simulink model "QuadcopterModel"  (R2023b)
settings: Solver=VariableStepAuto  StartTime=0.0  StopTime=200  RelTol=1e-3
values from neighbouring files (symbols this model uses):
  g = 9.81    [QuadcopterParameters.m]
  Ixx = 7.5e-3    (= 0.0075)    [QuadcopterParameters.m]
  Iyy = 7.5e-3    (= 0.0075)    [QuadcopterParameters.m]
  Izz = 1.3e-2    (= 0.013)    [QuadcopterParameters.m]
  Kf = 3.13e-5    (= 3.13e-05)    [QuadcopterParameters.m]
  Km = 7.5e-7    (= 7.5e-07)    [QuadcopterParameters.m]
  l = 0.23    [QuadcopterParameters.m]
  m = 0.65    [QuadcopterParameters.m]
  w1 = 200    [QuadcopterParameters.m]
  w2 = 200    [QuadcopterParameters.m]
  w3 = 10    [QuadcopterParameters.m]
  w4 = 10    [QuadcopterParameters.m]
undefined symbols (not defined in the file or in its folder): magnitude
settings Model: LastModifiedBy=DELL

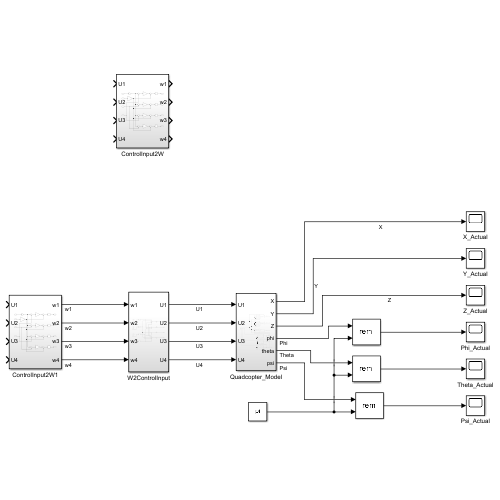
[thumbnail: Simulink's stored preview of the top-level diagram]
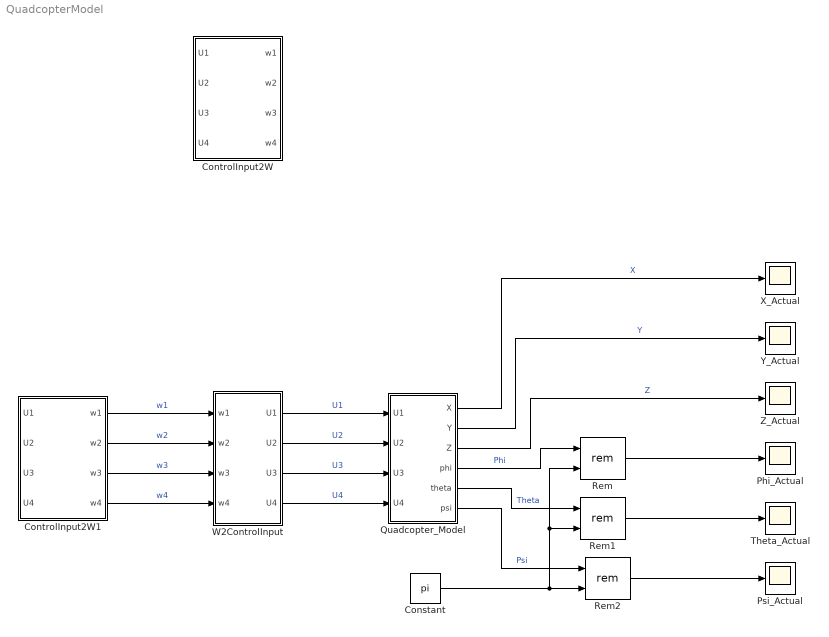
== system QuadcopterModel ==
  Constant : Constant  Value=pi
  ControlInput2W : Subsystem
  ControlInput2W1 : Subsystem
  Phi_Actual : Scope
  Psi_Actual : Scope
  Quadcopter_Model : Subsystem
  Rem : Math  Operator=rem
  Rem1 : Math  Operator=rem
  Rem2 : Math  Operator=rem
  Theta_Actual : Scope
  W2ControlInput : Subsystem
  X_Actual : Scope
  Y_Actual : Scope
  Z_Actual : Scope
  wires:
  W2ControlInput/1(U1) -> Quadcopter_Model/1(U1)  "U1"
  W2ControlInput/4(U4) -> Quadcopter_Model/4(U4)  "U4"
  Quadcopter_Model/3(Z) -> Z_Actual/1  "Z"
  Quadcopter_Model/2(Y) -> Y_Actual/1  "Y"
  Quadcopter_Model/1(X) -> X_Actual/1  "X"
  Constant/1 -> Rem2/2, Rem1/2, Rem/2
  Rem/1 -> Phi_Actual/1
  Rem1/1 -> Theta_Actual/1
  Rem2/1 -> Psi_Actual/1
  Quadcopter_Model/4(phi) -> Rem/1  "Phi"
  Quadcopter_Model/5(theta) -> Rem1/1  "Theta"
  Quadcopter_Model/6(psi) -> Rem2/1  "Psi"
  W2ControlInput/2(U2) -> Quadcopter_Model/2(U2)  "U2"
  W2ControlInput/3(U3) -> Quadcopter_Model/3(U3)  "U3"
  ControlInput2W1/1(w1) -> W2ControlInput/1(w1)  "w1"
  ControlInput2W1/2(w2) -> W2ControlInput/2(w2)  "w2"
  ControlInput2W1/3(w3) -> W2ControlInput/3(w3)  "w3"
  ControlInput2W1/4(w4) -> W2ControlInput/4(w4)  "w4"

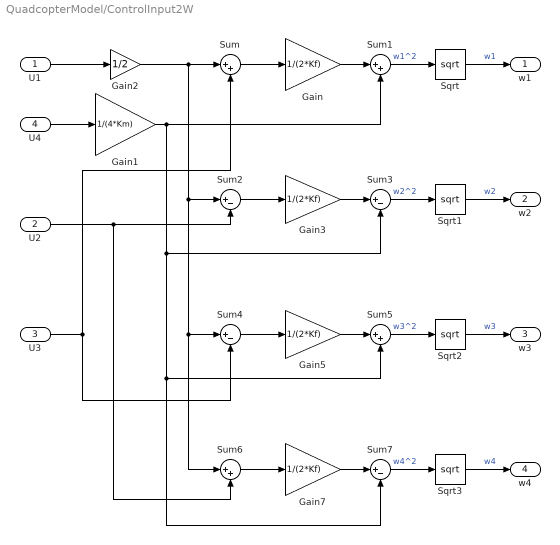
== system QuadcopterModel/ControlInput2W ==
  U1 : Inport
  U2 : Inport  Port=2
  U3 : Inport  Port=3
  U4 : Inport  Port=4
  Gain{,3,5,7} (4 alike) : Gain  Gain=1/(2*Kf)
  Gain1 : Gain  Gain=1/(4*Km)
  Gain2 : Gain  Gain=1/2
  Sqrt{,1..3} (4 alike) : Sqrt
  Sum{,1,5..6} (4 alike) : Sum  Inputs=|++
  Sum{2..4,7} (4 alike) : Sum  Inputs=|+-
  w1 : Outport
  w2 : Outport  Port=2
  w3 : Outport  Port=3
  w4 : Outport  Port=4
  wires:
  Sum7/1 -> Sqrt3/1  "w4^2"
  Gain5/1 -> Sum5/1
  Sum2/1 -> Gain3/1
  Gain/1 -> Sum1/1
  Gain3/1 -> Sum3/1
  Sqrt/1 -> w1/1  "w1"
  Gain7/1 -> Sum7/1
  Sum4/1 -> Gain5/1
  Sqrt1/1 -> w2/1  "w2"
  U2/1 -> Sum2/2, Sum6/2
  Sqrt2/1 -> w3/1  "w3"
  U1/1 -> Gain2/1
  Sqrt3/1 -> w4/1  "w4"
  Sum/1 -> Gain/1
  Gain2/1 -> Sum6/1, Sum4/1, Sum2/1, Sum/1
  Sum3/1 -> Sqrt1/1  "w2^2"
  U3/1 -> Sum/2, Sum4/2
  Sum6/1 -> Gain7/1
  Gain1/1 -> Sum3/2, Sum5/2, Sum7/2, Sum1/2
  Sum1/1 -> Sqrt/1  "w1^2"
  U4/1 -> Gain1/1
  Sum5/1 -> Sqrt2/1  "w3^2"

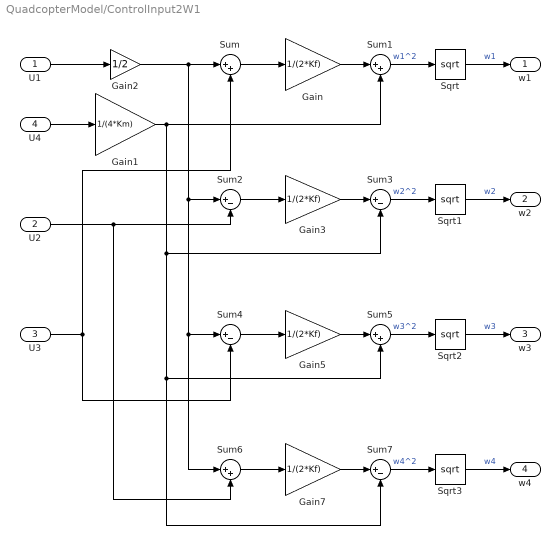
== system QuadcopterModel/ControlInput2W1 ==
  U1 : Inport
  U2 : Inport  Port=2
  U3 : Inport  Port=3
  U4 : Inport  Port=4
  Gain{,3,5,7} (4 alike) : Gain  Gain=1/(2*Kf)
  Gain1 : Gain  Gain=1/(4*Km)
  Gain2 : Gain  Gain=1/2
  Sqrt{,1..3} (4 alike) : Sqrt
  Sum{,1,5..6} (4 alike) : Sum  Inputs=|++
  Sum{2..4,7} (4 alike) : Sum  Inputs=|+-
  w1 : Outport
  w2 : Outport  Port=2
  w3 : Outport  Port=3
  w4 : Outport  Port=4
  wires:
  Sum7/1 -> Sqrt3/1  "w4^2"
  Gain5/1 -> Sum5/1
  Sum2/1 -> Gain3/1
  Gain/1 -> Sum1/1
  Gain3/1 -> Sum3/1
  Sqrt/1 -> w1/1  "w1"
  Gain7/1 -> Sum7/1
  Sum4/1 -> Gain5/1
  Sqrt1/1 -> w2/1  "w2"
  U2/1 -> Sum2/2, Sum6/2
  Sqrt2/1 -> w3/1  "w3"
  U1/1 -> Gain2/1
  Sqrt3/1 -> w4/1  "w4"
  Sum/1 -> Gain/1
  Gain2/1 -> Sum6/1, Sum4/1, Sum2/1, Sum/1
  Sum3/1 -> Sqrt1/1  "w2^2"
  U3/1 -> Sum/2, Sum4/2
  Sum6/1 -> Gain7/1
  Gain1/1 -> Sum3/2, Sum5/2, Sum7/2, Sum1/2
  Sum1/1 -> Sqrt/1  "w1^2"
  U4/1 -> Gain1/1
  Sum5/1 -> Sqrt2/1  "w3^2"

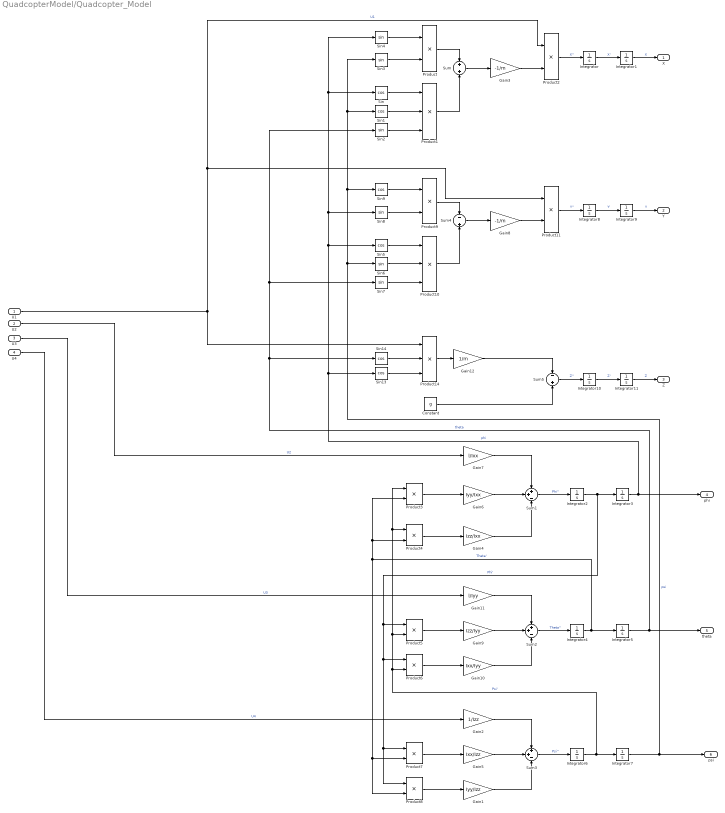
== system QuadcopterModel/Quadcopter_Model ==
  U1 : Inport
  U2 : Inport  Port=2
  U3 : Inport  Port=3
  U4 : Inport  Port=4
  Constant : Constant  Value=g
  Gain1 : Gain  Gain=Iyy/Izz
  Gain10 : Gain  Gain=Ixx/Iyy
  Gain11 : Gain  Gain=l/Iyy
  Gain12 : Gain  Gain=1/m
  Gain2 : Gain  Gain=1/Izz
  Gain3 : Gain  Gain=-1/m
  Gain4 : Gain  Gain=Izz/Ixx
  Gain5 : Gain  Gain=Ixx/Izz
  Gain6 : Gain  Gain=Iyy/Ixx
  Gain7 : Gain  Gain=l/Ixx
  Gain8 : Gain  Gain=-1/m
  Gain9 : Gain  Gain=Izz/Iyy
  Integrator{,1..11} (12 alike) : Integrator
  Product{,2..9,11} (10 alike) : Product
  Product1 : Product  Inputs=3
  Product10 : Product  Inputs=3
  Product14 : Product  Inputs=3
  Sin{,1,5,9,13..14} (6 alike) : Trigonometry  Operator=cos
  Sin{2..4,6..8} (6 alike) : Trigonometry
  Sum : Sum  Inputs=+|+
  Sum1 : Sum  Inputs=++-
  Sum2 : Sum  Inputs=++-
  Sum3 : Sum  Inputs=++-
  Sum4 : Sum  Inputs=-|+
  Sum5 : Sum  Inputs=-|+
  X : Outport
  Y : Outport  Port=2
  Z : Outport  Port=3
  phi : Outport  Port=4
  theta : Outport  Port=5
  psi : Outport  Port=6
  wires:
  Constant/1 -> Sum5/2
  Product2/1 -> Integrator/1  "X''"
  Sin7/1 -> Product10/3
  Product/1 -> Sum/1
  Integrator4/1 -> Integrator5/1, Product8/2, Product7/2, Product4/2, Product3/2  "Theta'"
  Sin9/1 -> Product9/1
  Gain8/1 -> Product11/2
  Sum/1 -> Gain3/1
  Product8/1 -> Gain1/1
  Sin4/1 -> Product/1
  Product5/1 -> Gain9/1
  Sum1/1 -> Integrator2/1  "Phi''"
  Sin5/1 -> Product10/1
  Gain11/1 -> Sum2/1
  Sin14/1 -> Product14/2
  Sin1/1 -> Product1/2
  Integrator/1 -> Integrator1/1  "X'"
  Integrator1/1 -> X/1  "X"
  Gain9/1 -> Sum2/2
  Integrator11/1 -> Z/1  "Z"
  Integrator3/1 -> phi/1, Sin8/1, Sin4/1, Sin/1, Sin5/1, Sin13/1  "phi"
  U3/1 -> Gain11/1  "U3"
  Product7/1 -> Gain5/1
  Integrator6/1 -> Product3/1, Product4/1, Product5/2, Product6/2, Integrator7/1  "Psi'"
  U1/1 -> Product2/1, Product11/1, Product14/1  "U1"
  Product14/1 -> Gain12/1
  Sum5/1 -> Integrator10/1  "Z''"
  Sin8/1 -> Product9/2
  Product4/1 -> Gain4/1
  Integrator7/1 -> Sin9/1, Sin3/1, Sin1/1, Sin6/1, psi/1  "psi"
  Sin2/1 -> Product1/3
  Product11/1 -> Integrator8/1  "Y''"
  Product3/1 -> Gain6/1
  Gain4/1 -> Sum1/3
  Gain5/1 -> Sum3/2
  Gain1/1 -> Sum3/3
  Sin/1 -> Product1/1
  Sum2/1 -> Integrator4/1  "Theta''"
  Gain3/1 -> Product2/2
  Gain10/1 -> Sum2/3
  Product9/1 -> Sum4/1
  Gain7/1 -> Sum1/1
  Sin6/1 -> Product10/2
  Sum3/1 -> Integrator6/1  "Psi''"
  Sum4/1 -> Gain8/1
  Gain6/1 -> Sum1/2
  Integrator8/1 -> Integrator9/1  "Y'"
  Gain12/1 -> Sum5/1
  Gain2/1 -> Sum3/1
  Product1/1 -> Sum/2
  Integrator9/1 -> Y/1  "Y"
  Integrator10/1 -> Integrator11/1  "Z'"
  Product6/1 -> Gain10/1
  Integrator5/1 -> theta/1, Sin14/1, Sin2/1, Sin7/1  "theta"
  Product10/1 -> Sum4/2
  U2/1 -> Gain7/1  "U2"
  Sin3/1 -> Product/2
  Integrator2/1 -> Product8/1, Product7/1, Product6/1, Product5/1, Integrator3/1  "Phi'"
  Sin13/1 -> Product14/3
  U4/1 -> Gain2/1  "U4"

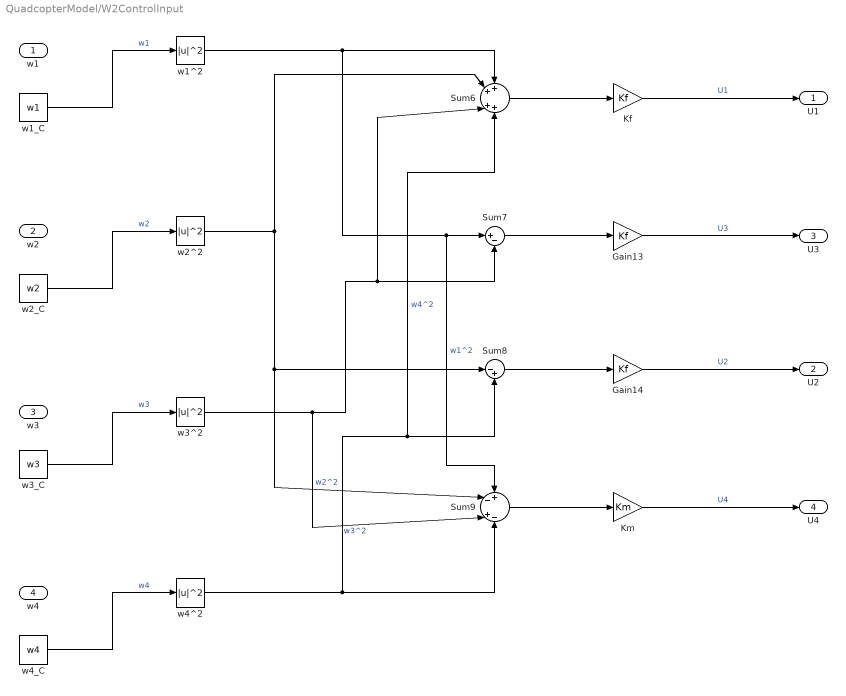
== system QuadcopterModel/W2ControlInput ==
  w1 : Inport
  w2 : Inport  Port=2
  w3 : Inport  Port=3
  w4 : Inport  Port=4
  Gain13 : Gain  Gain=Kf
  Gain14 : Gain  Gain=Kf
  Kf : Gain  Gain=Kf
  Km : Gain  Gain=Km
  Sum6 : Sum  Inputs=++|++
  Sum7 : Sum  Inputs=|+-
  Sum8 : Sum  Inputs=|-+
  Sum9 : Sum  Inputs=+-|+-
  w1^2 : Math  Operator=magnitude^2
  w1_C : Constant  Value=w1
  w2^2 : Math  Operator=magnitude^2
  w2_C : Constant  Value=w2
  w3^2 : Math  Operator=magnitude^2
  w3_C : Constant  Value=w3
  w4^2 : Math  Operator=magnitude^2
  w4_C : Constant  Value=w4
  U1 : Outport
  U2 : Outport  Port=2
  U3 : Outport  Port=3
  U4 : Outport  Port=4
  wires:
  Sum7/1 -> Gain13/1
  Sum6/1 -> Kf/1
  Sum8/1 -> Gain14/1
  Km/1 -> U4/1  "U4"
  w2^2/1 -> Sum6/2, Sum8/1, Sum9/2  "w2^2"
  Kf/1 -> U1/1  "U1"
  w4^2/1 -> Sum9/4, Sum8/2, Sum6/4  "w4^2"
  w1^2/1 -> Sum6/1, Sum9/1, Sum7/1  "w1^2"
  w3^2/1 -> Sum9/3, Sum6/3, Sum7/2  "w3^2"
  Gain14/1 -> U2/1  "U2"
  Gain13/1 -> U3/1  "U3"
  Sum9/1 -> Km/1
  w1_C/1 -> w1^2/1  "w1"
  w2_C/1 -> w2^2/1  "w2"
  w3_C/1 -> w3^2/1  "w3"
  w4_C/1 -> w4^2/1  "w4"
